simulink model "sim"  (R2018a)
settings: Solver=VariableStepAuto  StartTime=0.0  StopTime=10.0  RelTol=1e-3
settings Model: Creator=This PC  LastModifiedBy=This PC

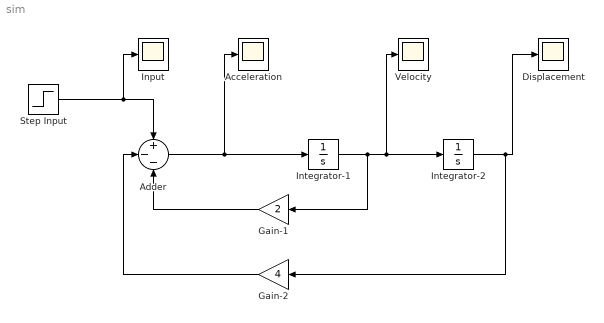
== system sim ==
  Acceleration : Scope
  Adder : Sum  Inputs=+--
  Displacement : Scope
  Gain-1 : Gain  Gain=2
  Gain-2 : Gain  Gain=4
  "Input " : Scope
  Integrator-1 : Integrator
  Integrator-2 : Integrator
  Step Input : Step  SampleTime=0
  Velocity : Scope
  wires:
  Step Input/1 -> "Input "/1, Adder/1
  Gain-1/1 -> Adder/3
  Gain-2/1 -> Adder/2
  Adder/1 -> Acceleration/1, Integrator-1/1
  Integrator-1/1 -> Gain-1/1, Velocity/1, Integrator-2/1
  Integrator-2/1 -> Gain-2/1, Displacement/1
